simulink model "Zad_2_szybkozmienny"  (R2018a)
settings: Solver=FixedStepAuto  StartTime=0.0  StopTime=0  RelTol=1e-3
libraries: CPOiS_SourcesSinks x4, CPOiS_DataManipulation x2, CPOiS_General x1
settings Model: Creator=rafal  LastModifiedBy=rafal

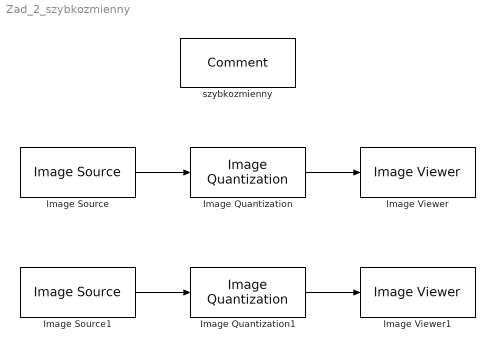
== system Zad_2_szybkozmienny ==
  Image Quantization : CPOiS_DataManipulation/Image Quantization  LevelsNum=32
      settings: SourceProductName=CPOiS - Digital image and signal processing
  Image Quantization1 : CPOiS_DataManipulation/Image Quantization  LevelsNum=4
      settings: SourceProductName=CPOiS - Digital image and signal processing
  Image Source : CPOiS_SourcesSinks/Image Source  FileSelection=gull.png
      settings: SourceProductName=CPOiS - Digital image and signal processing
  Image Source1 : CPOiS_SourcesSinks/Image Source  FileSelection=gull.png
      settings: SourceProductName=CPOiS - Digital image and signal processing
  Image Viewer : CPOiS_SourcesSinks/Image Viewer
      settings: SourceProductName=CPOiS - Digital image and signal processing
  Image Viewer1 : CPOiS_SourcesSinks/Image Viewer
      settings: SourceProductName=CPOiS - Digital image and signal processing
  "szybkozmienny " : CPOiS_General/Comment
      settings: SourceProductName=CPOiS - Digital image and signal processing
  wires:
  Image Quantization/1 -> Image Viewer/1
  Image Source1/1 -> Image Quantization1/1
  Image Quantization1/1 -> Image Viewer1/1
  Image Source/1 -> Image Quantization/1
